simulink library "simulink_extras"  (Simulink 7.5)
settings: Solver=ode45  SolverMode=SingleTasking  StartTime=0.0  StopTime=10.0  RelTol=1e-3
PostLoadFcn:
  | setsysloc simulink_extras
values from neighbouring files (symbols this model uses):
  A = [   zeros(q,1)    c ... (first row only)    [getxo.m]
  B = [  y - d * u ... (first row only)    [getxo.m]
  offset = block.DialogPrm(3).Data    [msfuncorr.m]    (also in msfunpsd.m = block.DialogPrm(4).Data; msfuntf.m = block.DialogPrm(4).Data)
undefined symbols (not defined in the file or in its folder): C, D, Dd, msfuncorr, msfunpsd
settings Model: Creator=ldean  LastModifiedBy=dyang  CovMetricSettings=d  ExtModeAutoUpdateStatusClock=off
settings Model: ForwardingTableString=|
  | ||__slOldName__||simulink_extras/Additional
  | Linear/PID Controller||__slNewName__||simulink_need_slupdate/PID Controller||__slOldName__||simulink_extras/Additional
  | Linear/PID Controller
  | (with Approximate
  | Derivative)||__slNewName__||simulink_need_slupdate/PID Controller
  | (with Approximate
  | Derivative)

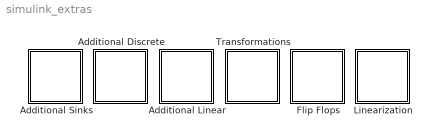
== system simulink_extras ==
  Additional Discrete : Subsystem
      mask Display: plot([-20 20],[-15 -15],[-15 -15],[-20 20], [ -15  -10  -10 -5 -5  0  0 5 5 10 10 15 15 20],[-10 -10 2  2  13 13 8  8  4  4  1  1  -1 -1])
  Additional Linear : Subsystem
      mask Display: plot([-20 20],[-15 -15],[-15 -15],[-20 20],[-20 20],[-5 18])
  Additional Sinks : Subsystem
      mask Display: plot([-1 1 1 -1 1],[ 1 -1 1 -1 1],[14 4 11 4 6],[14 4 6 4 11],[14 4 11 4 6],[-14 -4 -6 -4 -11],[-14 -4 -11 -4 -6],[14 4 6 4 11],[-14 -4 -11 -4 -6],[-14 -4 -6 -4 -11],[0 0 3 0 -3],[-20 -5 -10 -5 -10],[0 0 3 0 -3],[20 5 10 5 10],[20 5 10 5 10],[0 0 3 0 -3],[-20 -5 -10 -5 -10],[0 0 3 0 -3])
  Flip Flops : Subsystem
  Linearization : Subsystem
  Transformations : Subsystem

== system simulink_extras/Additional Discrete ==
  Discrete Transfer Fcn (with initial outputs) : Subsystem  mask(Discrete Transfer Function with Initial Outputs){N=[1], D=[1  .5], U0=[1], Y0=-.5, TS=1}
      mask prompts: N "Numerator:"; D "Denominator:"; U0 "Initial input:"; Y0 "Initial output:"; TS "Sample time:"
      mask help: Vector expressions for numerator, and denominator. Coefficients are in descending powers of z.
      mask init:
      | [A,B,C,Dd]=tf2ss(N,D);if (isempty(Y0));[m,n]=size(C);Y0=zeros(1,m); end;if (isempty(U0));[m,p]=size(B);U0=zeros(1,p);end;X0=getxo(A,B,C,Dd,U0,Y0,1);
      mask Help: Specify the initial output for the transfer function.  An optimization routine attempts to determine the appropriate initial states so that the specified initial output is achieved.  For more details, see the m-file getxo.m
      mask Display: dpoly(N,D,'z')
  Discrete Transfer Fcn (with initial states) : Subsystem  mask(Discrete Transfer Function with Initial States){N=[1], D=[1  .5], X0=[1], TS=.5}
      mask prompts: N "Numerator:"; D "Denominator:"; X0 "Initial conditions:"; TS "Sample time:"
      mask help: Vector expressions for numerator, and denominator. Coefficients are in descending powers of z.
      mask init:
      | [A,B,C,Dd]=tf2ss(N,D);if (isempty(X0));[m,n]=size(A);X0=zeros(1,m); end;
      mask Help: Specify the initial states for the transfer function.  The state ordering is determined by the m-file tf2ss.  There is no unique mapping of the states in a transfer function to states in a state-space representation.  However, tf2ss will consistently use the same mapping for a given transfer function.
      mask Display: dpoly(N,D,'z')
  Discrete Zero-Pole (with initial outputs) : Subsystem  mask(Discrete Zero-Pole with Initial Outputs){Z=[1], P=[0  .5], K=[1], U0=1, Y0=.5, TS=1}
      mask prompts: Z "Zeros:"; P "Poles:"; K "Gain:"; U0 "Initial input:"; Y0 "Initial output:"; TS "Sample time:"
      mask help: Vector expressions for numerator, denominator, and gain.
      mask init:
      | [A,B,C,D]=zp2ss(Z,P,K);if (isempty(Y0));[m,n]=size(C);Y0=zeros(1,m); end;if (isempty(U0));[m,p]=size(B);U0=zeros(1,p);end;X0=getxo(A,B,C,D,U0,Y0,1);
      mask Help: Specify the initial output for the zero-pole-gain system.  An optimization routine attempts to determine the appropriate initial states so that the specified initial output is achieved.  For more details, see the m-file getxo.m
      mask Display: droots(Z,P,K,'z')
  Discrete Zero-Pole (with initial states) : Subsystem  mask(Discrete Zero-Pole with Initial States){Z=[1], P=[0  .5], K=[1], X0=1, TS=.5}
      mask prompts: Z "Zeros:"; P "Poles:"; K "Gain:"; X0 "Initial conditions:"; TS "Sample time:"
      mask help: Vector expressions for numerator, denominator, and gain.
      mask init:
      | [A,B,C,D]=zp2ss(Z,P,K);if (isempty(X0));[m,n]=size(A);X0=zeros(1,m); end;
      mask Help: Specify the initial states for the transfer function.  The state ordering is determined by the m-file zp2ss.  There is no unique mapping of the states in a zero-pole-gain representation to states in a state-space representation.  However, zp2ss will consistently use the same mapping for a given transfer function.
      mask Display: droots(Z,P,K,'z')
  Idealized ADC quantizer : Subsystem  mask(IdealADC){NumberOfConverterBits=12, Vmin=0, Vmax=5, OutputDataType=int16, OutputNegativeValues=off}
      mask prompts: NumberOfConverterBits "Number of converter bits:"; Vmin "Min input voltage at low output:"; Vmax "Max input voltage at 2^n output (unreachable):"; OutputDataType "Output data type:"; OutputNegativeValues "Output negative values"
      mask help: Idealized quantizer for a linear analog to digital converter. There are 2^n possible digital output codes for an n-bit converter. Each value represents an equal fraction of the total analog input range in steps of one least significant bit (1 LSB). 1 LSB is (Vmax - Vmin)/2^bits. The midpoint of these steps corresponds to the actual value and thus introduce quantization error that is never more than 1/2 LSB within the full scale range (FSR). Since the first and last steps in the converter's range are only 1/2 LSB in width, the full scale range of the converter is equal to (2^n - 1) step widths. The FSR low transition occurs at Vmin + 1/2 LSB, the FSR high transition occurs at Vmax - 3/2 LSB. Conversion time is zero in this model. Set "Output negative values" to ON if you want negative outputs for negative voltages (does not apply to unsigned output data types).
      mask init:
      | blk = gcb;
      | set_param([blk,'/cast'], 'DataType', OutputDataType);
      | 
      | LSB    = (Vmax - Vmin) / pow2(NumberOfConverterBits);
      | invLSB =  pow2(NumberOfConverterBits) / (Vmax - Vmin);
      | 
      | if OutputNegativeValues ~= 0 && OutputDataType(1) ~= 'u'
      |     ZeroBias = -pow2(NumberOfConverterBits-1);
      | else
      | 	ZeroBias = 0;
      | end
      | 
      | % --- icon drawing data
      | 
      | b = 0.10;
      | m = 0.20;
      | steps_x = b + m*[0,0.5,0.5,1.5,1.5,2.5,2.5,3.5,4];
      | steps_y = b + m*[0,0,1,1,2,2,3,3,3];
      | line_xy = b + m*[0,4];
      settings: AttributesFormatString=(settings: %<NumberOfConverterBits>-bit converter\nVmin: %<Vmin>, Vmax: %<Vmax>)
      mask Help: Use this block to model an ideal analog to digital converter.  To model non-ideal converters, it is suggested to use a direct look-up table to represent static errors and dynamic models for transient error sources.  Use a discrete delay of the appropriate duration to model conversion latency if this is a significant value in your application.  If there is an input mux, model this with triggered latencies on the input side of the A/D block.
      mask StyleString: edit,edit,edit,popup(double|single|int8|uint8|int16|uint16|int32|uint32|boolean),checkbox
      mask Display:
      | plot(steps_x,steps_y)
      | plot(line_xy, line_xy)
      | port_label('input',1,'A')
      | port_label('output',1,'D')
      | text(0.5,0.9,[num2str(NumberOfConverterBits),' bits'],'horizontalalignment','center')

== system simulink_extras/Additional Linear ==
  State-Space (with initial outputs) : Subsystem  mask(State-Space with Initial Outputs){A=[-2.0479 -.4517;-.4517 -3.0295], B=[.0591 0]', C=[.2641 .8717], D=0, U0=1, Y0=.5}
      mask prompts: U0 "Initial inputs:"; Y0 "Initial outputs:"
      mask help:
      | State-Space model matrices:
      | dx/dt = Ax + Bu
      | y=Cx +Du
      mask init:
      | if (isempty(Y0));[m,n]=size(C);Y0=zeros(1,m); end; if (isempty(U0));[m,p]=size(B);U0=zeros(1,p);end;X0=getxo(A,B,C,D,U0,Y0,0);
      mask Help: Specify an initial output.  An optimization routine is used to attempt to find the steady state x values that satisfy the initial output.  The block states will be initialized to these values.
      mask Display: fprintf('x'' = Ax + Bu\n  y = Cx + Du');
  Transfer Fcn (with initial outputs) : Subsystem  mask(Transfer Function with Initial Outputs){N=[1], D=[1  1], Y0=.5, U0=0}
      mask prompts: N "Numerator:"; D "Denominator:"; Y0 "Initial output:"; U0 "Initial input:"
      mask help: Vector expressions for numerator, and denominator. Coefficients are in descending powers of s.
      mask init:
      | [A,B,C,Dd]=tf2ss(N,D);
      | if (isempty(Y0));
      |     [m,n]=size(C);
      |     Y0=zeros(1,m); 
      | end; 
      | if (isempty(U0));
      |     [m,p]=size(B);
      |     U0=zeros(1,p);
      | end;
      | X0=getxo(A,B,C,Dd,U0,Y0,0);
      mask Help: Specify the initial output for the transfer function.  An optimization routine attempts to determine the appropriate initial states so that the specified initial output is achieved.  For more details, see the m-file getxo.m
      mask Display: dpoly(N,D,'s')
  Transfer Fcn (with initial states) : Subsystem  mask(Transfer Function with Initial States){N=[1], D=[1  1], X0=.5}
      mask prompts: N "Numerator:"; D "Denominator:"; X0 "Initial conditions:"
      mask help: Vector expressions for numerator, and denominator. Coefficients are in descending powers of s.
      mask init:
      | [A,B,C,Dd]=tf2ss(N,D);if (isempty(X0));[m,n]=size(A);X0=zeros(1,m); end;
      mask Help: Specify the initial states for the transfer function.  The state ordering is determined by the m-file tf2ss.  There is no unique mapping of the states in a transfer function to states in a state-space representation.  However, tf2ss will consistently use the same mapping for a given transfer function.
      mask Display: dpoly(N,D,'s')
  Zero-Pole (with initial outputs) : Subsystem  mask(Zero-Pole with Initial Outputs){Z=[1], P=[0; -1], K=[1], Y0=.5, U0=0}
      mask prompts: Z "Zeros:"; P "Poles:"; K "Gain:"; Y0 "Initial output:"; U0 "Initial input:"
      mask help: Vector expressions for numerator, denominator, and gain.
      mask init:
      | [A,B,C,D]=zp2ss(Z,P,K);if (isempty(Y0));[m,n]=size(C);Y0=zeros(1,m); end; if (isempty(U0));[m,p]=size(B);U0=zeros(1,p);end;X0=getxo(A,B,C,D,U0,Y0,0);
      mask Help: Specify the initial output for the zero-pole-gain system.  An optimization routine attempts to determine the appropriate initial states so that the specified initial output is achieved.  For more details, see the m-file getxo.m
      mask Display: droots(Z,P,K)
  Zero-Pole (with initial states) : Subsystem  mask(Zero-Pole with Initial States){Z=[1], P=[0; -1], K=[1], X0=.5}
      mask prompts: Z "Zeros:"; P "Poles:"; K "Gain:"; X0 "Initial conditions:"
      mask help: Vector expressions for numerator, denominator, and gain.
      mask init:
      | [A,B,C,D]=zp2ss(Z,P,K);if (isempty(X0));[m,n]=size(A);X0=zeros(1,m); end;
      mask Help: Specify the initial states for the transfer function.  The state ordering is determined by the m-file zp2ss.  There is no unique mapping of the states in a zero-pole-gain representation to states in a state-space representation.  However, zp2ss will consistently use the same mapping for a given transfer function.
      mask Display: droots(Z,P,K)

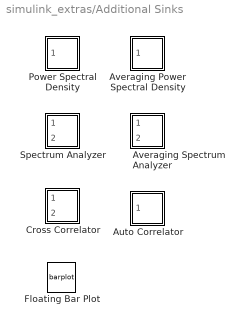
== system simulink_extras/Additional Sinks ==
  Auto Correlator : Subsystem  LoadFcn=msfuncorr([],'LoadBlock')  TreatAsAtomicUnit=on  SimViewingDevice=on  mask(Auto Correlator){npts=100, HowOften=50, sampleT=0.1}
      mask prompts: npts "Length of buffer:"; HowOften "Plot after how many points:"; sampleT "Sample time:"
      mask help:
      | Plots the auto correlation of the input.
      | Requires signal processing toolbox.
      mask init:
      | ts=sampleT(1); if length(sampleT) > 1, offset = sampleT(2); else offset = 0; end
      |  if HowOften > npts
      |     error('The number of points in the buffer must be more than the plot frequency')
      |  end
      settings: CopyFcn=msfuncorr([],'CopyBlock')  DeleteFcn=msfuncorr([],'DeleteBlock')  NameChangeFcn=msfuncorr([],'NameChange')
      mask Help: This block when hooked to the output of a system displays the auto correlation of the buffer in the graph window. For more see the M-file msfuncorr.
      mask Display: plot(0,0,100,100,[11,93,93,11,11],[90,90,40,40,90],[80,60,40,20],[50,79,50,80])
  Averaging Power Spectral Density : Subsystem  LoadFcn=msfunpsd([],'LoadBlock')  StartFcn=msfunpsd([],'Start')  TreatAsAtomicUnit=on  mask(Averaging Power Spectral Density){npts=128, fftpts=512, HowOften=64, sampleT=0.1}
      mask prompts: npts "Length of buffer:"; fftpts "Number of points for fft:"; HowOften "Plot after how many points:"; sampleT "Sample time:"
      mask help: Plots the averaged PSD of the input.
      mask init:
      | ts=sampleT(1); if length(sampleT) > 1, offset = sampleT(2); else offset = 0; end
      |  if HowOften > npts
      |     error('The number of points in the buffer must be more than the plot frequency')
      |  end
      settings: CopyFcn=msfunpsd([],'CopyBlock')  DeleteFcn=msfunpsd([],'DeleteBlock')  NameChangeFcn=msfunpsd([],'NameChange')
      mask Help: This block when hooked to the output of a system displays the frequency content of the buffer in the graph window. For more see the M-file msfunpsd.
      mask Display: plot(0,0,100,100,[11,92,92,11,11],[90,90,40,40,90],[82,76,65,57,51,44,35,30,25,20],[65,62,59,63,66,66,67,70,55,50])
  Averaging Spectrum Analyzer : Subsystem  TreatAsAtomicUnit=on  mask(Averaging Spectrum Analyzer){npts=256, fftpts=256, HowOften=64, sampleT=0.1}
      mask prompts: npts "Length of buffer:"; fftpts "Number of points for fft:"; HowOften "Plot after how many points:"; sampleT "Sample time:"
      mask help:
      | Implements an Averaging Spectrum analyzer.
      | Hook input 1 to system input.
      | Hook input 2 to system output.
      mask init:
      | ts=sampleT(1); if length(sampleT) > 1, offset = sampleT(2);, else, offset = 0; end
      mask Help: Hook the system's input to the first port of this block and the system's output to second port. Results are displayed as the frequency response of this system. Use signals with high harmonic content for best results.
      mask Display: plot(0,0,100,100,[12,92,92,12,12],[90,90,40,40,90],[80,72,63,54,47,40,32,20],[61,61,62,65,69,73,75,75])
  Cross Correlator : Subsystem  LoadFcn=msfuncorr([],'LoadBlock')  TreatAsAtomicUnit=on  SimViewingDevice=on  mask(Cross Correlator){npts=100, HowOften=50, sampleT=0.1}
      mask prompts: npts "Length of buffer:"; HowOften "Plot after how many points:"; sampleT "Sample time:"
      mask help:
      | Plots the cross correlation of the input signals.
      | Requires signal processing toolbox.
      mask init:
      | ts=sampleT(1); if length(sampleT) > 1, offset = sampleT(2);, else, offset = 0; end
      settings: CopyFcn=msfuncorr([],'CopyBlock')  DeleteFcn=msfuncorr([],'DeleteBlock')  NameChangeFcn=msfuncorr([],'NameChange')
      mask Help: This block when hooked to the outputs of a system displays the cross correlation of the buffer in the graph window. For more see the M-file msfuncorr.
      mask Display: plot(0,0,100,100,[10,92,92,10,10],[90,90,40,40,90],[80,59,40,20],[70,79,70,79],[79,70,59,51,40,30,21],[60,51,60,50,60,50,60])
  Floating Bar Plot : S-Function  FunctionName=barplot  Parameters=yLim  EnableBusSupport=off  mask(Floating Bar Plot){yLim=[-6 6  -5 5  -5 5  -5 5  -5 5  -5 5  -5 5  -5 5  -5 5  -5 5  -5 5]}
      mask prompts: yLim "Y-Limits"
      mask help: Displays selected signals as bar plot while the simulation is running (i.e., click on signal lines to see their values displayed). To select multiple signals use shift-click. Each signal is displayed in its own axes, using the corresponding set of Y-Limits.
      mask init:
      | x=[0.1 0.1 0.2 0.2 0.3 0.3 0.4 0.4 0.5 0.5 0.6 0.6 0.7 0.7 0.8 0.8 0.1];
      | y=[0.0 0.6 0.6 0.0 0.0 0.8 0.8 0.0 0.0 0.9 0.9 0.0 0.0 0.4 0.4 0.0 0.0];
      settings: DeleteFcn=barplotm([],'DeleteFcn')  NameChangeFcn=barplotm([],'NameChangeFcn')
      mask Help: Displays selected signal values (click on signal) as bar plot while the simulation is running.  To select multiple signals use shift-click.  Each signal (selected line) is displayed in it's own axes.  The 1stY-Limits pair is used for the 1st axes, the 2nd for the 2nd axes, etc.   If there are more axes, than Y-Limits pairs, the last Y-Limits pair is used.
      mask Display: plot(x,y);
  Power Spectral Density : Subsystem  LoadFcn=msfunpsd([],'LoadBlock')  StartFcn=msfunpsd([],'Start')  TreatAsAtomicUnit=on  mask(Power Spectral Density){npts=128, fftpts=512, HowOften=64, sampleT=0.1}
      mask prompts: npts "Length of buffer:"; fftpts "Number of points for fft:"; HowOften "Plot after how many points:"; sampleT "Sample time:"
      mask help: Plot the PSD of the input.
      mask init:
      | ts=sampleT(1); if length(sampleT) > 1, offset = sampleT(2);, else, offset = 0; end
      settings: CopyFcn=msfunpsd([],'CopyBlock')  DeleteFcn=msfunpsd([],'DeleteBlock')  NameChangeFcn=msfunpsd([],'NameChange')
      mask Help: This block when hooked to the output of a system displays the frequency content of the buffer in the graph window. For more see the M-file msfunpsd.
      mask Display: plot(0,0,100,100,[14,91,91,14,14],[86,86,40,40,86],[85,82,80,79,75,67,63,60,57,53,41,36,33,27,24],[49,50,53,50,49,51,54,66,54,50,50,52,81,51,49])
  Spectrum Analyzer : Subsystem  TreatAsAtomicUnit=on  mask(Spectrum Analyzer){npts=256, fftpts=256, HowOften=64, sampleT=0.1}
      mask prompts: npts "Length of buffer:"; fftpts "Number of points for fft:"; HowOften "Plot after how many points:"; sampleT "Sample time:"
      mask help:
      | Implements a Spectrum Analyzer.
      | Hook input 1 to system input.
      | Hook input 2 to system output.
      mask init:
      | ts=sampleT(1); if length(sampleT) > 1, offset = sampleT(2);, else, offset = 0; end
      mask Help: Hook the system's input to the first port of this block and the system's output to second port. Results are displayed as the frequency response of this system. Use signals with high harmonic content for best results.
      mask Display: plot(0,0,100,100,[11,93,93,11,11],[90,90,40,40,90],[90,80,72,64,55,45,41,36,20],[50,50,52,59,67,75,78,80,80])

== system simulink_extras/Flip Flops ==
  note: Note: J-K Flip-Flop is Negative-Edge-Triggered
  Clock : Subsystem  mask(Digital clock){period=2}
      mask help:
      | Digital clock.
      | Output is set to 1 for the first half of the period.
      mask init:
      | duration = period/2;
      mask Help: web([docroot '/toolbox/simulink/ref_extras/clock.html'])
      mask Display: plot(0,0,100,100,[90,75,75,60,60,35,35,20,20,10],[20,20,80,80,19,20,80,80,20,20])
  D Flip-Flop : Subsystem
      mask Type: DFlipFlop
      mask Description: D Flip-Flop Block
      mask Help: web([docroot '/toolbox/simulink/ref_extras/dflipflop.html'])
  D Latch : Subsystem
      mask Type: DLatch
      mask Description: D Latch Flip-Flop Block
      mask Help: web([docroot '/toolbox/simulink/ref_extras/dlatch.html'])
  J-K Flip-Flop : Subsystem  mask(JKFlipFlop){initial_condition=0}
      mask prompts: initial_condition "Initial condition (state of Q):"
      mask help: J-K Flip-Flop Block (Negative Edge Triggered)
      mask Help: web([docroot '/toolbox/simulink/ref_extras/jkflipflop.html'])
  S-R Flip-Flop : Subsystem  mask(SRFlipFlop){initial_condition=0}
      mask prompts: initial_condition "Initial condition (state of Q):"
      mask help: S-R Flip-Flop Block
      mask Help: web([docroot '/toolbox/simulink/ref_extras/srflipflop.html'])

== system simulink_extras/Linearization ==
  note: Block for use with linmod:
  Switched derivative for linearization : Subsystem  mask(Derivative for linearization){switchVal=0, derivConst=100}
      mask prompts: switchVal "Switch value (1 for linearization, 0 for simulation):"; derivConst "Derivative constant  Ns/(s+N):"
      mask help: Switched derivative with proper transfer function approximation for linearization.
      mask init:
      | num = [derivConst,0]; den = [1, derivConst];
      mask Help: This block should be used in place of the derivative when you are linearizing the model. It approximates the derivative with a proper transfer function.
      mask Display: disp('du/dt')
  Switched transport delay for linearization : TransportDelay  PadeOrder=2

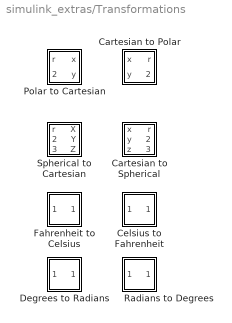
== system simulink_extras/Transformations ==
  Cartesian to Polar : Subsystem
      mask Type: Cart2Polar
      mask Description:
      | Transformation from cartesian to polar coordinates.
      | [x, y] -> [r, theta]
      | 
      | r = sqrt(x^2 + y^2);
      | theta = atan(y/x);
      mask Help: web([docroot '/toolbox/simulink/ref_extras/cartesiantopolar.html'])
      mask Display: plot(0,0,100,100,[24,20,15,20,20],[85,95,85,95,20],[80,20,95,85,95,85],[70,20,20,15,20,24],[56,56,55,52,50,46],[20,26,31,35,38,42])
  Cartesian to Spherical : Subsystem
      mask Type: Cart2Sph
      mask Description:
      | Transformation from cartesian to spherical coordinates.
      | [x, y, z] -> [r, theta, phi]
      | 
      | p = hypot(x,y); r = hypot(p,z);
      | theta = atan(y/x);
      | phi = atan(p/z);
      mask Help: web([docroot '/toolbox/simulink/ref_extras/cartesiantospherical.html'])
      mask Display: plot(0,0,100,100,[45,40,35,40,40],[85,95,85,95,30],[22,10,14,10,40,95,85,95,85],[12,10,20,10,30,30,25,30,35],[70,40],[80,30],[54,52,50,47,44,40],[53,55,56,58,59,59])
  Celsius to Fahrenheit : Subsystem
      mask Type: CelsiusToFahrenheit
      mask Description:
      | Conversion from degrees Celsius to degrees Fahrenheit.
      | 
      | F=9/5*C+32
      mask Help: web([docroot '/toolbox/simulink/ref_extras/celsiustofahrenheit.html'])
      mask Display: disp('C2F')
  Degrees to Radians : Subsystem
      mask Type: DegreesToRadians
      mask Description:
      | Conversion from Degrees to Radians.
      | 
      | R=pi/180*D
      mask Help: web([docroot '/toolbox/simulink/ref_extras/degreestoradians.html'])
      mask Display: disp('D2R')
  Fahrenheit to Celsius : Subsystem
      mask Type: FahrenheitToCelsius
      mask Description:
      | Conversion from degrees Fahrenheit to degrees Celsius.
      | 
      | C=5/9*(F-32);
      mask Help: web([docroot '/toolbox/simulink/ref_extras/fahrenheittocelsius.html'])
      mask Display: disp('F2C')
  Polar to Cartesian : Subsystem
      mask Type: Polar2Cart
      mask Description:
      | Transformation from polar to cartesian coordinates.
      | [r, theta] -> [x, y]
      | 
      | x = r * cos(theta);
      | y = r * sin(theta);
      mask Help: web([docroot '/toolbox/simulink/ref_extras/polartocartesian.html'])
      mask Display: plot(0,0,100,100,[25,20,15,20,20],[85,95,85,95,20],[70,20,95,86,95,85],[60,20,20,15,20,25],[70,70],[45,54],[70,70],[30,40],[70,70],[20,25],[55,65],[60,60],[40,50],[60,60],[25,34],[60,60],[20,21],[60,60],[70,70,68],[57,60,60])
  Radians to Degrees : Subsystem
      mask Type: RadiansToDegrees
      mask Description:
      | Conversion from Radians to Degrees.
      | 
      | D=180/pi*R
      mask Help: web([docroot '/toolbox/simulink/ref_extras/radianstodegrees.html'])
      mask Display: disp('R2D')
  Spherical to Cartesian : Subsystem
      mask Type: Sph2Cart
      mask Description:
      | Transformation from spherical to cartesian coordinates.
      | [r, theta, phi] -> [x, y, z]
      | 
      | x = r * sin(phi) * cos(theta);
      | y = r * sin(phi) * sin(theta);
      | z = r * cos(phi);
      mask Help: web([docroot '/toolbox/simulink/ref_extras/sphericaltocartesian.html'])
      mask Display: plot(0,0,100,100,[45,40,35,40,40],[85,95,85,95,40],[85,95,85,95,40],[35,40,45,40,40],[60,40,10,20,10,14],[70,40,10,13,10,20],[56,45],[70,70],[60,60],[50,60],[60,60],[30,40],[50,60],[20,20],[30,40],[20,20],[45,55],[35,25],[75,65],[35,25])

== system simulink_extras/Additional Discrete/Discrete Transfer Fcn (with initial outputs) ==
  In1 : Inport  OutDataType=sfix(16)  OutScaling=2^0
  Discrete State Space : DiscreteStateSpace  A=A  B=B  C=C  D=Dd  X0=X0  SampleTime=TS
  Out1 : Outport  OutDataType=sfix(16)  OutScaling=2^0  InitialOutput=0
  wires:
  Discrete State Space/1 -> Out1/1
  In1/1 -> Discrete State Space/1

== system simulink_extras/Additional Discrete/Discrete Transfer Fcn (with initial states) ==
  In1 : Inport  OutDataType=sfix(16)  OutScaling=2^0
  Discrete State Space : DiscreteStateSpace  A=A  B=B  C=C  D=Dd  X0=X0  SampleTime=TS
  Out1 : Outport  OutDataType=sfix(16)  OutScaling=2^0  InitialOutput=0
  wires:
  Discrete State Space/1 -> Out1/1
  In1/1 -> Discrete State Space/1

== system simulink_extras/Additional Discrete/Discrete Zero-Pole (with initial outputs) ==
  In1 : Inport  OutDataType=sfix(16)  OutScaling=2^0
  Discrete State Space : DiscreteStateSpace  A=A  B=B  C=C  D=D  X0=X0  SampleTime=TS
  Out1 : Outport  OutDataType=sfix(16)  OutScaling=2^0  InitialOutput=0
  wires:
  Discrete State Space/1 -> Out1/1
  In1/1 -> Discrete State Space/1

== system simulink_extras/Additional Discrete/Discrete Zero-Pole (with initial states) ==
  In1 : Inport  OutDataType=sfix(16)  OutScaling=2^0
  Discrete State Space : DiscreteStateSpace  A=A  B=B  C=C  D=D  X0=X0  SampleTime=TS
  Out1 : Outport  OutDataType=sfix(16)  OutScaling=2^0  InitialOutput=0
  wires:
  Discrete State Space/1 -> Out1/1
  In1/1 -> Discrete State Space/1

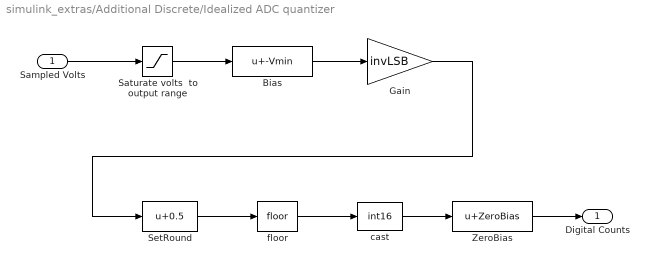
== system simulink_extras/Additional Discrete/Idealized ADC quantizer ==
  Sampled Volts : Inport  OutDataType=sfix(16)  OutScaling=2^0
  Bias : Bias  Bias=-Vmin
  Gain : Gain  Gain=invLSB  ParameterDataType=sfix(16)  ParameterScaling=2^0  OutDataType=sfix(16)  OutScaling=2^0
  Saturate volts  to output range : Saturate  UpperLimit=Vmax - (LSB*3/2)  LowerLimit=Vmin  OutDataType=sfix(16)  OutScaling=2^0
      settings: AttributesFormatString=Max = %<UpperLimit>\nMin = %<LowerLimit>
  SetRound : Bias  Bias=0.5
  ZeroBias : Bias  Bias=ZeroBias
  cast : DataTypeConversion  OutDataTypeMode=int16  OutDataType=sfix(16)  OutScaling=2^0  OutDataTypeStr=int16  RndMeth=Zero
  floor : Rounding
  Digital Counts : Outport  OutDataType=sfix(16)  OutScaling=2^0
  wires:
  Sampled Volts/1 -> Saturate volts  to output range/1
  cast/1 -> ZeroBias/1
  SetRound/1 -> floor/1
  floor/1 -> cast/1
  Saturate volts  to output range/1 -> Bias/1
  Gain/1 -> SetRound/1
  Bias/1 -> Gain/1
  ZeroBias/1 -> Digital Counts/1

== system simulink_extras/Additional Linear/State-Space (with initial outputs) ==
  In1 : Inport  OutDataType=sfix(16)  OutScaling=2^0
  State-Space : StateSpace  A=A  B=B  C=C  D=D  X0=X0
  Out1 : Outport  OutDataType=sfix(16)  OutScaling=2^0  InitialOutput=0
  wires:
  In1/1 -> State-Space/1
  State-Space/1 -> Out1/1

== system simulink_extras/Additional Linear/Transfer Fcn (with initial outputs) ==
  In1 : Inport  OutDataType=sfix(16)  OutScaling=2^0
  State Space : StateSpace  A=A  B=B  C=C  D=Dd  X0=X0
  Out1 : Outport  OutDataType=sfix(16)  OutScaling=2^0  InitialOutput=0
  wires:
  In1/1 -> State Space/1
  State Space/1 -> Out1/1

== system simulink_extras/Additional Linear/Transfer Fcn (with initial states) ==
  In1 : Inport  OutDataType=sfix(16)  OutScaling=2^0
  State Space : StateSpace  A=A  B=B  C=C  D=Dd  X0=X0
  Out1 : Outport  OutDataType=sfix(16)  OutScaling=2^0  InitialOutput=0
  wires:
  In1/1 -> State Space/1
  State Space/1 -> Out1/1

== system simulink_extras/Additional Linear/Zero-Pole (with initial outputs) ==
  In1 : Inport  OutDataType=sfix(16)  OutScaling=2^0
  State Space : StateSpace  A=A  B=B  C=C  D=D  X0=X0
  Out1 : Outport  OutDataType=sfix(16)  OutScaling=2^0  InitialOutput=0
  wires:
  In1/1 -> State Space/1
  State Space/1 -> Out1/1

== system simulink_extras/Additional Linear/Zero-Pole (with initial states) ==
  In1 : Inport  OutDataType=sfix(16)  OutScaling=2^0
  State Space : StateSpace  A=A  B=B  C=C  D=D  X0=X0
  Out1 : Outport  OutDataType=sfix(16)  OutScaling=2^0  InitialOutput=0
  wires:
  In1/1 -> State Space/1
  State Space/1 -> Out1/1

== system simulink_extras/Additional Sinks/Auto Correlator ==
  input signal : Inport  OutDataType=sfix(16)  OutScaling=2^0
  msfuncorr : M-S-Function  FunctionName=msfuncorr  Parameters=npts,HowOften,offset,ts,0,'unbiased'
  wires:
  input signal/1 -> msfuncorr/1

== system simulink_extras/Additional Sinks/Averaging Power Spectral Density ==
  input signal : Inport  OutDataType=sfix(16)  OutScaling=2^0
  msfunpsd : M-S-Function  FunctionName=msfunpsd  Parameters=fftpts,npts,HowOften,offset,ts,1
  wires:
  input signal/1 -> msfunpsd/1

== system simulink_extras/Additional Sinks/Averaging Spectrum Analyzer ==
  system input : Inport  OutDataType=sfix(16)  OutScaling=2^0
  system output : Inport  Port=2  OutDataType=sfix(16)  OutScaling=2^0
  Mux : Mux  Inputs=2
  msfuntf : M-S-Function  FunctionName=msfuntf  Parameters=fftpts,npts,HowOften,offset,ts,1
  wires:
  Mux/1 -> msfuntf/1
  system input/1 -> Mux/1
  system output/1 -> Mux/2

== system simulink_extras/Additional Sinks/Cross Correlator ==
  signal 1 : Inport  OutDataType=sfix(16)  OutScaling=2^0
  signal 2 : Inport  Port=2  OutDataType=sfix(16)  OutScaling=2^0
  Mux : Mux  Inputs=2
  msfuncorr : M-S-Function  FunctionName=msfuncorr  Parameters=npts,HowOften,offset,ts,1,'unbiased'
  wires:
  signal 1/1 -> Mux/1
  signal 2/1 -> Mux/2
  Mux/1 -> msfuncorr/1

== system simulink_extras/Additional Sinks/Power Spectral Density ==
  input signal : Inport  OutDataType=sfix(16)  OutScaling=2^0
  msfunpsd : M-S-Function  FunctionName=msfunpsd  Parameters=fftpts,npts,HowOften,offset,ts,0
  wires:
  input signal/1 -> msfunpsd/1

== system simulink_extras/Additional Sinks/Spectrum Analyzer ==
  system input : Inport  OutDataType=sfix(16)  OutScaling=2^0
  system output : Inport  Port=2  OutDataType=sfix(16)  OutScaling=2^0
  Mux : Mux  Inputs=2
  msfuntf : M-S-Function  FunctionName=msfuntf  Parameters=fftpts,npts,HowOften,offset,ts,0
  wires:
  system output/1 -> Mux/2
  system input/1 -> Mux/1
  Mux/1 -> msfuntf/1

== system simulink_extras/Flip Flops/Clock ==
  Constant : Constant  OutDataType=sfix(16)  OutScaling=2^0
  Sum : Sum  Inputs=+-  OutDataType=sfix(16)  OutScaling=2^0  SaturateOnIntegerOverflow=on  InputSameDT=on  OutDataTypeStr=Inherit: Same as first input
  Unit Delay : UnitDelay  SampleTime=duration
  out_1 : Outport  OutDataType=sfix(16)  OutScaling=2^0  InitialOutput=0
  wires:
  Unit Delay/1 -> Sum/2
  Sum/1 -> out_1/1, Unit Delay/1
  Constant/1 -> Sum/1

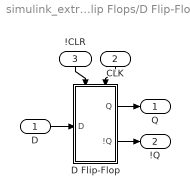
== system simulink_extras/Flip Flops/D Flip-Flop ==
  D : Inport  OutDataType=sfix(16)  OutScaling=2^0
  CLK : Inport  Port=2  OutDataType=sfix(16)  OutScaling=2^0
  !CLR : Inport  Port=3  OutDataType=sfix(16)  OutScaling=2^0
  D Flip-Flop : Subsystem  TreatAsAtomicUnit=on
  Q : Outport  OutDataType=sfix(16)  OutScaling=2^0  InitialOutput=0
  !Q : Outport  Port=2  OutDataType=sfix(16)  OutScaling=2^0  InitialOutput=1
  wires:
  CLK/1 -> D Flip-Flop/Trigger
  !CLR/1 -> D Flip-Flop/Enable
  D Flip-Flop/1(Q) -> Q/1
  D/1 -> D Flip-Flop/1(D)
  D Flip-Flop/2(!Q) -> !Q/1

== system simulink_extras/Flip Flops/D Latch ==
  D : Inport  OutDataType=sfix(16)  OutScaling=2^0
  C : Inport  Port=2  OutDataType=sfix(16)  OutScaling=2^0
  D Latch : Subsystem  TreatAsAtomicUnit=on
  Q : Outport  OutDataType=sfix(16)  OutScaling=2^0  InitialOutput=0
  !Q : Outport  Port=2  OutDataType=sfix(16)  OutScaling=2^0  InitialOutput=1
  wires:
  D Latch/2(!Q) -> !Q/1
  D/1 -> D Latch/1(D)
  D Latch/1(Q) -> Q/1
  C/1 -> D Latch/Enable

== system simulink_extras/Flip Flops/J-K Flip-Flop ==
  J : Inport  OutDataType=sfix(16)  OutScaling=2^0
  CLK : Inport  Port=2  OutDataType=sfix(16)  OutScaling=2^0
  K : Inport  Port=3  OutDataType=sfix(16)  OutScaling=2^0
  J-K Flip-Flop : Subsystem  TreatAsAtomicUnit=on
  Q : Outport  OutDataType=sfix(16)  OutScaling=2^0
  !Q : Outport  Port=2  OutDataType=sfix(16)  OutScaling=2^0
  wires:
  J-K Flip-Flop/2(!Q) -> !Q/1
  K/1 -> J-K Flip-Flop/2(K)
  J/1 -> J-K Flip-Flop/1(J)
  J-K Flip-Flop/1(Q) -> Q/1
  CLK/1 -> J-K Flip-Flop/Trigger

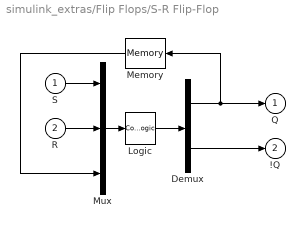
== system simulink_extras/Flip Flops/S-R Flip-Flop ==
  S : Inport  OutDataType=sfix(16)  OutScaling=2^0
  R : Inport  Port=2  OutDataType=sfix(16)  OutScaling=2^0
  Demux : Demux  Outputs=2
  Logic : CombinatorialLogic  TruthTable=[0 1;1 0;0 1;0 1;1 0;1 0;0 0;0 0]
  Memory : Memory  X0=initial_condition  InheritSampleTime=on
  Mux : Mux  Inputs=3
  Q : Outport  OutDataType=sfix(16)  OutScaling=2^0  InitialOutput=0
  !Q : Outport  Port=2  OutDataType=sfix(16)  OutScaling=2^0  InitialOutput=1
  wires:
  R/1 -> Mux/2
  S/1 -> Mux/1
  Demux/1 -> Memory/1, Q/1
  Demux/2 -> !Q/1
  Logic/1 -> Demux/1
  Mux/1 -> Logic/1
  Memory/1 -> Mux/3

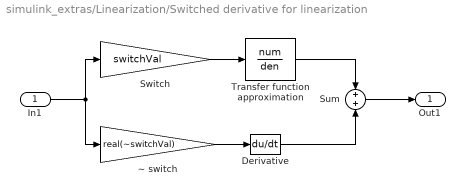
== system simulink_extras/Linearization/Switched derivative for linearization ==
  In1 : Inport  OutDataType=sfix(16)  OutScaling=2^0
  Derivative : Derivative
  Sum : Sum  OutDataType=sfix(16)  OutScaling=2^0  SaturateOnIntegerOverflow=on  InputSameDT=on  OutDataTypeStr=Inherit: Same as first input
  Switch : Gain  Gain=switchVal  ParameterDataType=sfix(16)  ParameterScaling=2^0  OutDataType=sfix(16)  OutScaling=2^0  SaturateOnIntegerOverflow=on  OutDataTypeStr=Inherit: Same as input  ParamDataTypeStr=Inherit: Same as input
  Transfer function approximation : TransferFcn  Numerator=num  Denominator=den
  ~ switch : Gain  Gain=real(~switchVal)  ParameterDataType=sfix(16)  ParameterScaling=2^0  OutDataType=sfix(16)  OutScaling=2^0  SaturateOnIntegerOverflow=on  OutDataTypeStr=Inherit: Same as input  ParamDataTypeStr=Inherit: Same as input
  Out1 : Outport  OutDataType=sfix(16)  OutScaling=2^0
  wires:
  In1/1 -> ~ switch/1, Switch/1
  Switch/1 -> Transfer function approximation/1
  ~ switch/1 -> Derivative/1
  Derivative/1 -> Sum/2
  Transfer function approximation/1 -> Sum/1
  Sum/1 -> Out1/1

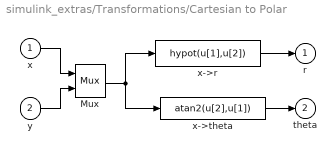
== system simulink_extras/Transformations/Cartesian to Polar ==
  x : Inport  PortDimensions=1  OutDataType=sfix(16)  OutScaling=2^0
  y : Inport  Port=2  PortDimensions=1  OutDataType=sfix(16)  OutScaling=2^0
  Mux : Mux  Inputs=2
  x->r : Fcn  Expr=hypot(u[1],u[2])
  x->theta : Fcn  Expr=atan2(u[2],u[1])
  r : Outport  OutDataType=sfix(16)  OutScaling=2^0  InitialOutput=0
  theta : Outport  Port=2  OutDataType=sfix(16)  OutScaling=2^0  InitialOutput=0
  wires:
  x->theta/1 -> theta/1
  y/1 -> Mux/2
  x/1 -> Mux/1
  x->r/1 -> r/1
  Mux/1 -> x->r/1, x->theta/1

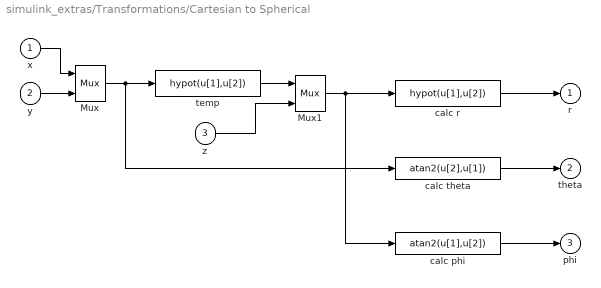
== system simulink_extras/Transformations/Cartesian to Spherical ==
  x : Inport  PortDimensions=1  OutDataType=sfix(16)  OutScaling=2^0
  y : Inport  Port=2  PortDimensions=1  OutDataType=sfix(16)  OutScaling=2^0
  z : Inport  Port=3  PortDimensions=1  OutDataType=sfix(16)  OutScaling=2^0
  Mux : Mux  Inputs=2
  Mux1 : Mux  Inputs=2
  calc phi : Fcn  Expr=atan2(u[1],u[2])
  calc r : Fcn  Expr=hypot(u[1],u[2])
  calc theta : Fcn  Expr=atan2(u[2],u[1])
  temp : Fcn  Expr=hypot(u[1],u[2])
  "r " : Outport  OutDataType=sfix(16)  OutScaling=2^0  InitialOutput=0
  theta : Outport  Port=2  OutDataType=sfix(16)  OutScaling=2^0  InitialOutput=0
  phi : Outport  Port=3  OutDataType=sfix(16)  OutScaling=2^0  InitialOutput=0
  wires:
  Mux1/1 -> calc r/1, calc phi/1
  Mux/1 -> temp/1, calc theta/1
  calc r/1 -> "r "/1
  z/1 -> Mux1/2
  temp/1 -> Mux1/1
  x/1 -> Mux/1
  y/1 -> Mux/2
  calc phi/1 -> phi/1
  calc theta/1 -> theta/1

== system simulink_extras/Transformations/Celsius to Fahrenheit ==
  Celsius in : Inport  OutDataType=sfix(16)  OutScaling=2^0
  Constant : Constant  Value=32  OutDataType=sfix(16)  OutScaling=2^0  OutDataTypeStr=Inherit: Inherit via back propagation
  Gain : Gain  Gain=9/5  ParameterDataType=sfix(16)  ParameterScaling=2^0  OutDataType=sfix(16)  OutScaling=2^0  SaturateOnIntegerOverflow=on  OutDataTypeStr=Inherit: Same as input  ParamDataTypeStr=Inherit: Same as input
  Sum : Sum  OutDataType=sfix(16)  OutScaling=2^0  SaturateOnIntegerOverflow=on  InputSameDT=on  OutDataTypeStr=Inherit: Same as first input
  Fahrenheit out : Outport  OutDataType=sfix(16)  OutScaling=2^0  InitialOutput=0
  wires:
  Constant/1 -> Sum/2
  Sum/1 -> Fahrenheit out/1
  Gain/1 -> Sum/1
  Celsius in/1 -> Gain/1

== system simulink_extras/Transformations/Degrees to Radians ==
  Degrees in : Inport  OutDataType=sfix(16)  OutScaling=2^0
  Gain1 : Gain  Gain=pi/180  ParameterDataType=sfix(16)  ParameterScaling=2^0  OutDataType=sfix(16)  OutScaling=2^0  SaturateOnIntegerOverflow=on  OutDataTypeStr=Inherit: Same as input  ParamDataTypeStr=Inherit: Same as input
  Radians out : Outport  OutDataType=sfix(16)  OutScaling=2^0  InitialOutput=0
  wires:
  Degrees in/1 -> Gain1/1
  Gain1/1 -> Radians out/1

== system simulink_extras/Transformations/Fahrenheit to Celsius ==
  Fahrenheit in : Inport  OutDataType=sfix(16)  OutScaling=2^0
  Constant : Constant  Value=32  OutDataType=sfix(16)  OutScaling=2^0  OutDataTypeStr=Inherit: Inherit via back propagation
  Gain1 : Gain  Gain=5/9  ParameterDataType=sfix(16)  ParameterScaling=2^0  OutDataType=sfix(16)  OutScaling=2^0  SaturateOnIntegerOverflow=on  OutDataTypeStr=Inherit: Same as input  ParamDataTypeStr=Inherit: Same as input
  Sum : Sum  Inputs=+-  OutDataType=sfix(16)  OutScaling=2^0  SaturateOnIntegerOverflow=on  InputSameDT=on  OutDataTypeStr=Inherit: Same as first input
  Celsius out : Outport  OutDataType=sfix(16)  OutScaling=2^0  InitialOutput=0
  wires:
  Gain1/1 -> Celsius out/1
  Sum/1 -> Gain1/1
  Fahrenheit in/1 -> Sum/1
  Constant/1 -> Sum/2

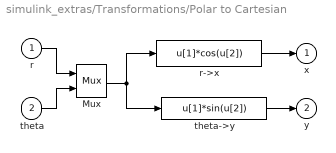
== system simulink_extras/Transformations/Polar to Cartesian ==
  "r " : Inport  PortDimensions=1  OutDataType=sfix(16)  OutScaling=2^0
  "theta " : Inport  Port=2  PortDimensions=1  OutDataType=sfix(16)  OutScaling=2^0
  Mux : Mux  Inputs=2
  r->x : Fcn  Expr=u[1]*cos(u[2])
  theta->y : Fcn  Expr=u[1]*sin(u[2])
  x : Outport  OutDataType=sfix(16)  OutScaling=2^0  InitialOutput=0
  y : Outport  Port=2  OutDataType=sfix(16)  OutScaling=2^0  InitialOutput=0
  wires:
  Mux/1 -> r->x/1, theta->y/1
  r->x/1 -> x/1
  "r "/1 -> Mux/1
  "theta "/1 -> Mux/2
  theta->y/1 -> y/1

== system simulink_extras/Transformations/Radians to Degrees ==
  Radians in : Inport  OutDataType=sfix(16)  OutScaling=2^0
  Gain : Gain  Gain=180/pi  ParameterDataType=sfix(16)  ParameterScaling=2^0  OutDataType=sfix(16)  OutScaling=2^0  SaturateOnIntegerOverflow=on  OutDataTypeStr=Inherit: Same as input  ParamDataTypeStr=Inherit: Same as input
  Degrees out : Outport  OutDataType=sfix(16)  OutScaling=2^0  InitialOutput=0
  wires:
  Radians in/1 -> Gain/1
  Gain/1 -> Degrees out/1

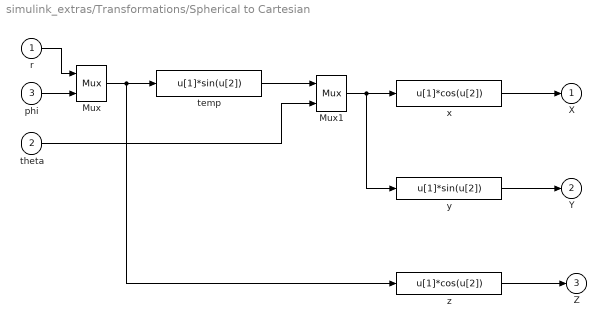
== system simulink_extras/Transformations/Spherical to Cartesian ==
  r : Inport  PortDimensions=1  OutDataType=sfix(16)  OutScaling=2^0
  theta : Inport  Port=2  PortDimensions=1  OutDataType=sfix(16)  OutScaling=2^0
  phi : Inport  Port=3  PortDimensions=1  OutDataType=sfix(16)  OutScaling=2^0
  Mux : Mux  Inputs=2
  Mux1 : Mux  Inputs=2
  temp : Fcn  Expr=u[1]*sin(u[2])
  x : Fcn  Expr=u[1]*cos(u[2])
  y : Fcn  Expr=u[1]*sin(u[2])
  z : Fcn  Expr=u[1]*cos(u[2])
  X : Outport  OutDataType=sfix(16)  OutScaling=2^0  InitialOutput=0
  Y : Outport  Port=2  OutDataType=sfix(16)  OutScaling=2^0  InitialOutput=0
  Z : Outport  Port=3  OutDataType=sfix(16)  OutScaling=2^0  InitialOutput=0
  wires:
  Mux/1 -> temp/1, z/1
  Mux1/1 -> x/1, y/1
  theta/1 -> Mux1/2
  phi/1 -> Mux/2
  r/1 -> Mux/1
  temp/1 -> Mux1/1
  x/1 -> X/1
  y/1 -> Y/1
  z/1 -> Z/1

== system simulink_extras/Flip Flops/D Flip-Flop/D Flip-Flop ==
  D : Inport  OutDataType=sfix(16)  OutScaling=2^0  LatchByDelayingOutsideSignal=on
  C : EnablePort
  Trigger : TriggerPort  StatesWhenEnabling=reset
  Logic : Logic  Operator=NOT  Inputs=1
  Q : Outport  OutDataType=sfix(16)  OutScaling=2^0  OutputWhenDisabled=reset  InitialOutput=0
  !Q : Outport  Port=2  OutDataType=sfix(16)  OutScaling=2^0  OutputWhenDisabled=reset  InitialOutput=1
  wires:
  Logic/1 -> !Q/1
  D/1 -> Q/1, Logic/1

== system simulink_extras/Flip Flops/D Latch/D Latch ==
  D : Inport  OutDataType=sfix(16)  OutScaling=2^0
  C : EnablePort
  Logic : Logic  Operator=NOT  Inputs=1
  Q : Outport  OutDataType=sfix(16)  OutScaling=2^0  InitialOutput=0
  !Q : Outport  Port=2  OutDataType=sfix(16)  OutScaling=2^0  InitialOutput=1
  wires:
  D/1 -> Logic/1, Q/1
  Logic/1 -> !Q/1

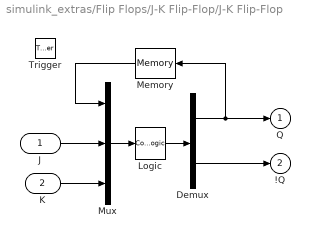
== system simulink_extras/Flip Flops/J-K Flip-Flop/J-K Flip-Flop ==
  J : Inport  OutDataType=sfix(16)  OutScaling=2^0  LatchByDelayingOutsideSignal=on
  K : Inport  Port=2  OutDataType=sfix(16)  OutScaling=2^0  LatchByDelayingOutsideSignal=on
  Trigger : TriggerPort  TriggerType=falling  StatesWhenEnabling=reset
  Demux : Demux  Outputs=2
  Logic : CombinatorialLogic  TruthTable=[0 1; 0 1; 1 0; 1 0; 1 0; 0 1; 1 0; 0 1]
  Memory : Memory  X0=initial_condition  InheritSampleTime=on
  Mux : Mux  Inputs=3
  Q : Outport  OutDataType=sfix(16)  OutScaling=2^0  InitialOutput=initial_condition
  !Q : Outport  Port=2  OutDataType=sfix(16)  OutScaling=2^0  InitialOutput=~initial_condition
  wires:
  J/1 -> Mux/2
  K/1 -> Mux/3
  Memory/1 -> Mux/1
  Demux/1 -> Q/1, Memory/1
  Demux/2 -> !Q/1
  Logic/1 -> Demux/1
  Mux/1 -> Logic/1
